simulink model "lab3_p9"  (R2020a)
settings: Solver=VariableStepAuto  StartTime=0.0  StopTime=mp.test_signal.duration  RelTol=1e-3
InitFcn:
  | sm_callback_init
StopFcn:
  | sm_callback_stop
values from neighbouring files (symbols this model uses):
  mp = sm_init_control_signals(mp)    [sm_callback_init.m]    (also in sm_callback_stop.m = sm_stop_verify(mp))
undefined symbols (not defined in the file or in its folder): magnitude
libraries: hdlsllib x9, simulink x3
settings Model: Creator=Owner  LastModifiedBy=Owner
settings DataIOCC: ReturnWorkspaceOutputs=off

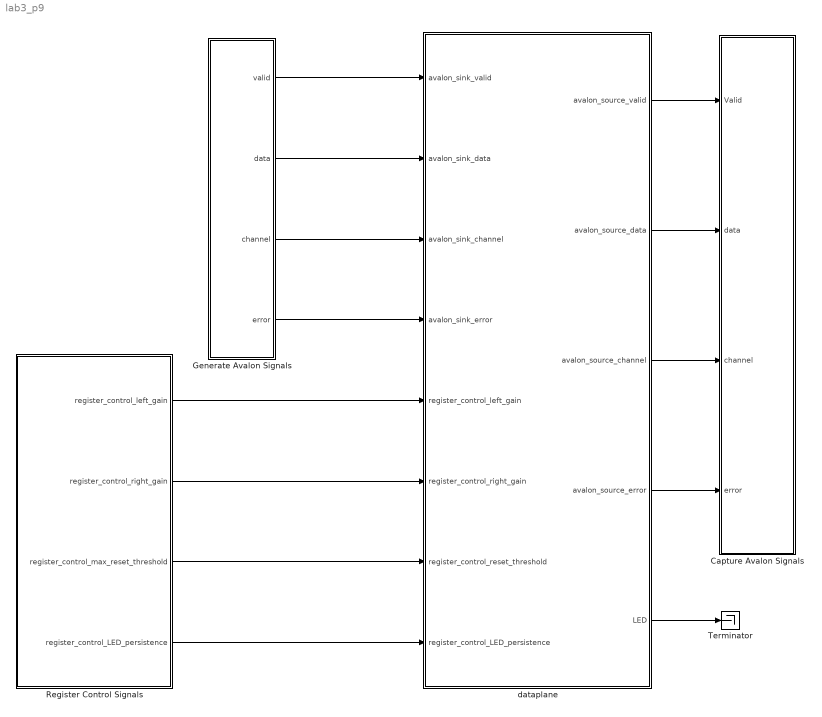
== system lab3_p9 ==
  Capture Avalon Signals : Subsystem
  Generate Avalon Signals : Subsystem
  Register Control Signals : Subsystem
  Terminator : Terminator
  dataplane : Subsystem
  wires:
  Generate Avalon Signals/1(valid) -> dataplane/1(avalon_sink_valid)
  Generate Avalon Signals/2(data) -> dataplane/2(avalon_sink_data)
  Generate Avalon Signals/3(channel) -> dataplane/3(avalon_sink_channel)
  Generate Avalon Signals/4(error) -> dataplane/4(avalon_sink_error)
  dataplane/1(avalon_source_valid) -> Capture Avalon Signals/1(Valid)
  dataplane/2(avalon_source_data) -> Capture Avalon Signals/2(data)
  dataplane/3(avalon_source_channel) -> Capture Avalon Signals/3(channel)
  dataplane/4(avalon_source_error) -> Capture Avalon Signals/4(error)
  Register Control Signals/2(register_control_right_gain) -> dataplane/6(register_control_right_gain)
  Register Control Signals/1(register_control_left_gain) -> dataplane/5(register_control_left_gain)
  Register Control Signals/3(register_control_max_reset_threshold) -> dataplane/7(register_control_reset_threshold)
  Register Control Signals/4(register_control_LED_persistence) -> dataplane/8(register_control_LED_persistence)
  dataplane/5(LED) -> Terminator/1

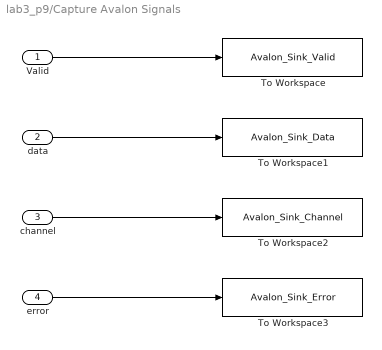
== system lab3_p9/Capture Avalon Signals ==
  Valid : Inport
  data : Inport  Port=2
  channel : Inport  Port=3
  error : Inport  Port=4
  To Workspace : ToWorkspace  VariableName=Avalon_Sink_Valid  SampleTime=-1
      settings: Save2DSignal=2-D array (concatenate along first dimension)
  To Workspace1 : ToWorkspace  VariableName=Avalon_Sink_Data  SampleTime=-1
      settings: Save2DSignal=2-D array (concatenate along first dimension)
  To Workspace2 : ToWorkspace  VariableName=Avalon_Sink_Channel  SampleTime=-1
      settings: Save2DSignal=2-D array (concatenate along first dimension)
  To Workspace3 : ToWorkspace  VariableName=Avalon_Sink_Error  SampleTime=-1
      settings: Save2DSignal=2-D array (concatenate along first dimension)
  wires:
  Valid/1 -> To Workspace/1
  data/1 -> To Workspace1/1
  channel/1 -> To Workspace2/1
  error/1 -> To Workspace3/1

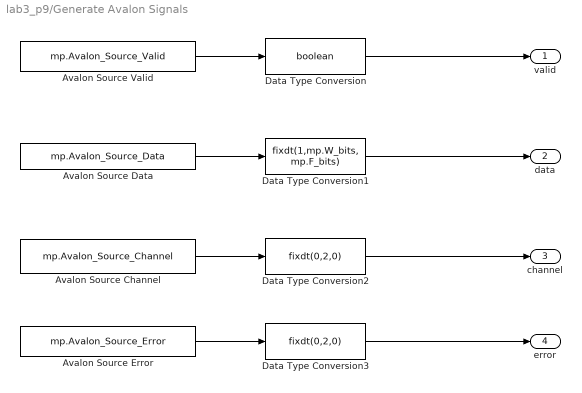
== system lab3_p9/Generate Avalon Signals ==
  Avalon Source Channel : FromWorkspace  VariableName=mp.Avalon_Source_Channel  OutDataTypeStr=double  SampleTime=mp.Ts_system
  Avalon Source Data : FromWorkspace  VariableName=mp.Avalon_Source_Data  OutDataTypeStr=double  SampleTime=mp.Ts_system
  Avalon Source Error : FromWorkspace  VariableName=mp.Avalon_Source_Error  OutDataTypeStr=double  SampleTime=mp.Ts_system
  Avalon Source Valid : FromWorkspace  VariableName=mp.Avalon_Source_Valid  OutDataTypeStr=double  SampleTime=mp.Ts_system
  Data Type Conversion : DataTypeConversion  OutDataTypeStr=boolean  RndMeth=Nearest
  Data Type Conversion1 : DataTypeConversion  OutDataTypeStr=fixdt(1,mp.W_bits, mp.F_bits)  RndMeth=Nearest
  Data Type Conversion2 : DataTypeConversion  OutDataTypeStr=fixdt(0,2,0)  RndMeth=Nearest
  Data Type Conversion3 : DataTypeConversion  OutDataTypeStr=fixdt(0,2,0)  RndMeth=Nearest
  valid : Outport
  data : Outport  Port=2
  channel : Outport  Port=3
  error : Outport  Port=4
  wires:
  Data Type Conversion/1 -> valid/1
  Avalon Source Valid/1 -> Data Type Conversion/1
  Avalon Source Data/1 -> Data Type Conversion1/1
  Data Type Conversion1/1 -> data/1
  Data Type Conversion2/1 -> channel/1
  Avalon Source Channel/1 -> Data Type Conversion2/1
  Data Type Conversion3/1 -> error/1
  Avalon Source Error/1 -> Data Type Conversion3/1

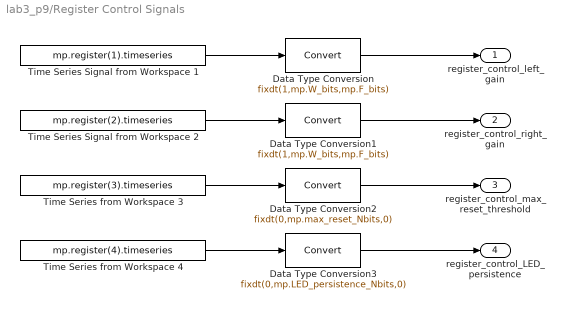
== system lab3_p9/Register Control Signals ==
  Data Type Conversion : DataTypeConversion  OutDataTypeStr=fixdt(1,mp.W_bits,mp.F_bits)
  Data Type Conversion1 : DataTypeConversion  OutDataTypeStr=fixdt(1,mp.W_bits,mp.F_bits)
  Data Type Conversion2 : DataTypeConversion  OutDataTypeStr=fixdt(0,mp.max_reset_Nbits,0)
  Data Type Conversion3 : DataTypeConversion  OutDataTypeStr=fixdt(0,mp.LED_persistence_Nbits,0)
  Time Series Signal from Workspace 1 : FromWorkspace  VariableName=mp.register(1).timeseries  OutDataTypeStr=double  SampleTime=mp.Ts_system
  Time Series Signal from Workspace 2 : FromWorkspace  VariableName=mp.register(2).timeseries  OutDataTypeStr=double  SampleTime=mp.Ts_system
  Time Series from Workspace 3 : FromWorkspace  VariableName=mp.register(3).timeseries  OutDataTypeStr=double  SampleTime=mp.Ts_system
  Time Series from Workspace 4 : FromWorkspace  VariableName=mp.register(4).timeseries  OutDataTypeStr=double  SampleTime=mp.Ts_system
  register_control_left_gain : Outport
  register_control_right_gain : Outport  Port=2
  register_control_max_reset_threshold : Outport  Port=3
  register_control_LED_persistence : Outport  Port=4
  wires:
  Time Series Signal from Workspace 1/1 -> Data Type Conversion/1
  Data Type Conversion/1 -> register_control_left_gain/1
  Time Series Signal from Workspace 2/1 -> Data Type Conversion1/1
  Data Type Conversion1/1 -> register_control_right_gain/1
  Data Type Conversion2/1 -> register_control_max_reset_threshold/1
  Data Type Conversion3/1 -> register_control_LED_persistence/1
  Time Series from Workspace 4/1 -> Data Type Conversion3/1
  Time Series from Workspace 3/1 -> Data Type Conversion2/1

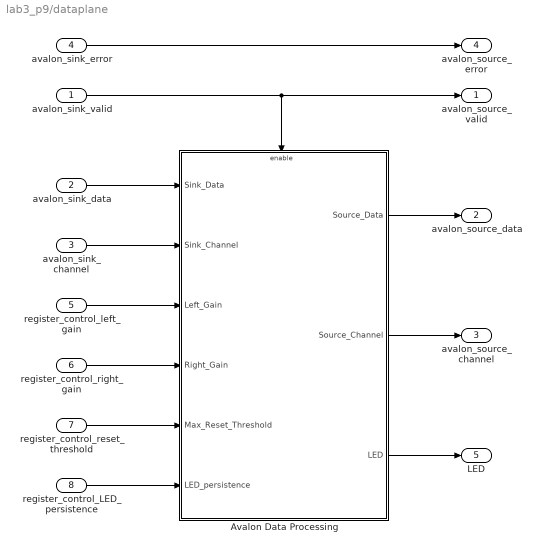
== system lab3_p9/dataplane ==
  avalon_sink_valid : Inport
  avalon_sink_data : Inport  Port=2
  avalon_sink_channel : Inport  Port=3
  avalon_sink_error : Inport  Port=4
  register_control_left_gain : Inport  Port=5
  register_control_right_gain : Inport  Port=6
  register_control_reset_threshold : Inport  Port=7
  register_control_LED_persistence : Inport  Port=8
  Avalon Data Processing : Subsystem  TreatAsAtomicUnit=on
  avalon_source_valid : Outport  VectorParamsAs1DForOutWhenUnconnected=off
  avalon_source_data : Outport  Port=2  VectorParamsAs1DForOutWhenUnconnected=off
  avalon_source_channel : Outport  Port=3  VectorParamsAs1DForOutWhenUnconnected=off
  avalon_source_error : Outport  Port=4  VectorParamsAs1DForOutWhenUnconnected=off
  LED : Outport  Port=5  VectorParamsAs1DForOutWhenUnconnected=off
  wires:
  avalon_sink_error/1 -> avalon_source_error/1
  avalon_sink_valid/1 -> avalon_source_valid/1, Avalon Data Processing/Enable
  Avalon Data Processing/1(Source_Data) -> avalon_source_data/1
  Avalon Data Processing/2(Source_Channel) -> avalon_source_channel/1
  avalon_sink_data/1 -> Avalon Data Processing/1(Sink_Data)
  avalon_sink_channel/1 -> Avalon Data Processing/2(Sink_Channel)
  register_control_right_gain/1 -> Avalon Data Processing/4(Right_Gain)
  register_control_left_gain/1 -> Avalon Data Processing/3(Left_Gain)
  register_control_reset_threshold/1 -> Avalon Data Processing/5(Max_Reset_Threshold)
  register_control_LED_persistence/1 -> Avalon Data Processing/6(LED_persistence)
  Avalon Data Processing/3(LED) -> LED/1

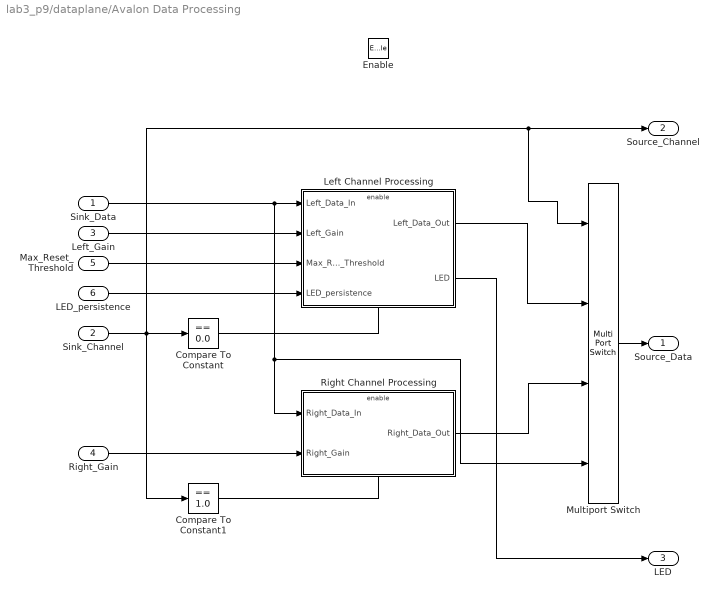
== system lab3_p9/dataplane/Avalon Data Processing ==
  Sink_Data : Inport
  Sink_Channel : Inport  Port=2
  Left_Gain : Inport  Port=3
  Right_Gain : Inport  Port=4
  Max_Reset_Threshold : Inport  Port=5
  LED_persistence : Inport  Port=6
  Enable : EnablePort
  Compare To Constant : simulink/Logic and Bit Operations/Compare To Constant  relop===  const=0.0  OutDataTypeStr=boolean
  Compare To Constant1 : simulink/Logic and Bit Operations/Compare To Constant  relop===  const=1.0  OutDataTypeStr=boolean
  Left Channel Processing : Subsystem  TreatAsAtomicUnit=on
  Multiport Switch : MultiPortSwitch  DataPortOrder=Zero-based contiguous  zeroidx=on
  Right Channel Processing : Subsystem  TreatAsAtomicUnit=on
  Source_Data : Outport
  Source_Channel : Outport  Port=2
  LED : Outport  Port=3
  wires:
  Sink_Data/1 -> Multiport Switch/4, Right Channel Processing/1(Right_Data_In), Left Channel Processing/1(Left_Data_In)
  Sink_Channel/1 -> Compare To Constant1/1, Multiport Switch/1, Source_Channel/1, Compare To Constant/1
  Left_Gain/1 -> Left Channel Processing/2(Left_Gain)
  Right_Gain/1 -> Right Channel Processing/2(Right_Gain)
  Compare To Constant1/1 -> Right Channel Processing/Enable
  Compare To Constant/1 -> Left Channel Processing/Enable
  Multiport Switch/1 -> Source_Data/1
  Left Channel Processing/1(Left_Data_Out) -> Multiport Switch/2
  Right Channel Processing/1(Right_Data_Out) -> Multiport Switch/3
  Left Channel Processing/2(LED) -> LED/1
  LED_persistence/1 -> Left Channel Processing/4(LED_persistence)
  Max_Reset_Threshold/1 -> Left Channel Processing/3(Max_Reset_Threshold)

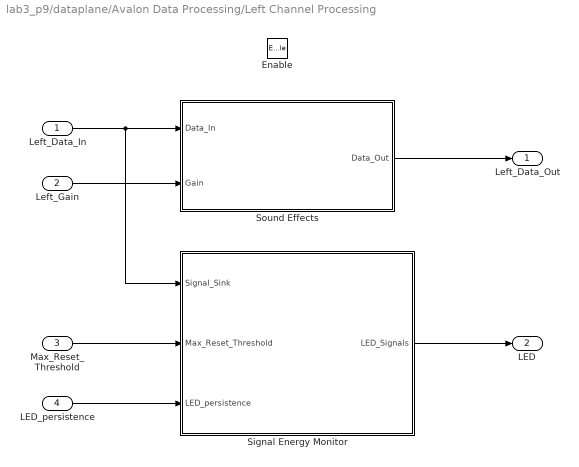
== system lab3_p9/dataplane/Avalon Data Processing/Left Channel Processing ==
  Left_Data_In : Inport
  Left_Gain : Inport  Port=2
  Max_Reset_Threshold : Inport  Port=3
  LED_persistence : Inport  Port=4
  Enable : EnablePort
  Signal Energy Monitor : Subsystem
  Sound Effects : Subsystem
  Left_Data_Out : Outport  InitialOutput=0  VectorParamsAs1DForOutWhenUnconnected=off
  LED : Outport  Port=2  InitialOutput=0  VectorParamsAs1DForOutWhenUnconnected=off
  wires:
  Sound Effects/1(Data_Out) -> Left_Data_Out/1
  Left_Gain/1 -> Sound Effects/2(Gain)
  Signal Energy Monitor/1(LED_Signals) -> LED/1
  LED_persistence/1 -> Signal Energy Monitor/3(LED_persistence)
  Left_Data_In/1 -> Signal Energy Monitor/1(Signal_Sink), Sound Effects/1(Data_In)
  Max_Reset_Threshold/1 -> Signal Energy Monitor/2(Max_Reset_Threshold)

== system lab3_p9/dataplane/Avalon Data Processing/Right Channel Processing ==
  Right_Data_In : Inport
  Right_Gain : Inport  Port=2
  Enable : EnablePort
  Sound Effects : Subsystem
  Right_Data_Out : Outport  InitialOutput=0  VectorParamsAs1DForOutWhenUnconnected=off
  wires:
  Right_Data_In/1 -> Sound Effects/1(Data_In)
  Right_Gain/1 -> Sound Effects/2(Gain)
  Sound Effects/1(Data_Out) -> Right_Data_Out/1

== system lab3_p9/dataplane/Avalon Data Processing/Left Channel Processing/Signal Energy Monitor ==
  Signal_Sink : Inport
  Max_Reset_Threshold : Inport  Port=2
  LED_persistence : Inport  Port=3
  LED_Driver : Subsystem
  Normalize Signal : Subsystem
  LED_Signals : Outport  VectorParamsAs1DForOutWhenUnconnected=off
  wires:
  Signal_Sink/1 -> Normalize Signal/1(Signal_Sink)
  Max_Reset_Threshold/1 -> Normalize Signal/2(Max_Reset_Threshold)
  Normalize Signal/1(Normalized_Signal_Energy) -> LED_Driver/1(Normalized_Signal)
  LED_Driver/1(LED_Signals) -> LED_Signals/1
  LED_persistence/1 -> LED_Driver/2(LED_persistence)

== system lab3_p9/dataplane/Avalon Data Processing/Left Channel Processing/Sound Effects ==
  Data_In : Inport
  Gain : Inport  Port=2
  Data Type Conversion : DataTypeConversion  OutDataTypeStr=fixdt(1,mp.W_bits,mp.F_bits)  RndMeth=Nearest
  Product : Product
  Data_Out : Outport
  wires:
  Product/1 -> Data Type Conversion/1
  Gain/1 -> Product/2
  Data_In/1 -> Product/1
  Data Type Conversion/1 -> Data_Out/1

== system lab3_p9/dataplane/Avalon Data Processing/Right Channel Processing/Sound Effects ==
  Data_In : Inport
  Gain : Inport  Port=2
  Data Type Conversion : DataTypeConversion  OutDataTypeStr=fixdt(1,mp.W_bits,mp.F_bits)  RndMeth=Nearest
  Product : Product
  Data_Out : Outport
  wires:
  Product/1 -> Data Type Conversion/1
  Gain/1 -> Product/2
  Data_In/1 -> Product/1
  Data Type Conversion/1 -> Data_Out/1

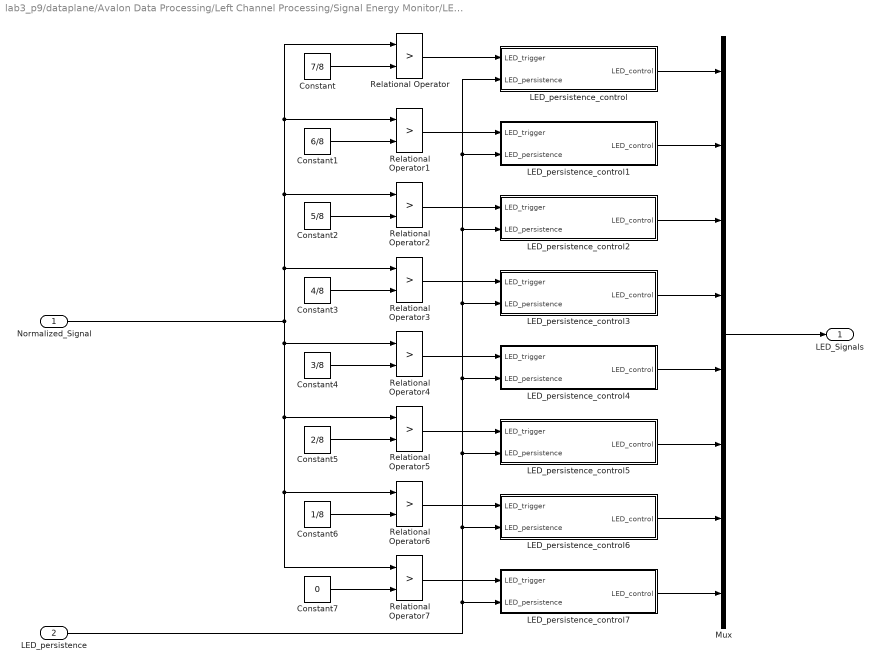
== system lab3_p9/dataplane/Avalon Data Processing/Left Channel Processing/Signal Energy Monitor/LED_Driver ==
  Normalized_Signal : Inport
  LED_persistence : Inport  Port=2
  Constant : Constant  Value=7/8  OutDataTypeStr=fixdt(1,mp.W_bits,mp.F_bits)  SampleTime=mp.Ts_system
  Constant1 : Constant  Value=6/8  OutDataTypeStr=fixdt(1,mp.W_bits,mp.F_bits)  SampleTime=mp.Ts_system
  Constant2 : Constant  Value=5/8  OutDataTypeStr=fixdt(1,mp.W_bits,mp.F_bits)  SampleTime=mp.Ts_system
  Constant3 : Constant  Value=4/8  OutDataTypeStr=fixdt(1,mp.W_bits,mp.F_bits)  SampleTime=mp.Ts_system
  Constant4 : Constant  Value=3/8  OutDataTypeStr=fixdt(1,mp.W_bits,mp.F_bits)  SampleTime=mp.Ts_system
  Constant5 : Constant  Value=2/8  OutDataTypeStr=fixdt(1,mp.W_bits,mp.F_bits)  SampleTime=mp.Ts_system
  Constant6 : Constant  Value=1/8  OutDataTypeStr=fixdt(1,mp.W_bits,mp.F_bits)  SampleTime=mp.Ts_system
  Constant7 : Constant  Value=0  OutDataTypeStr=fixdt(1,mp.W_bits,mp.F_bits)  SampleTime=mp.Ts_system
  LED_persistence_control : Subsystem
  LED_persistence_control1 : Subsystem
  LED_persistence_control2 : Subsystem
  LED_persistence_control3 : Subsystem
  LED_persistence_control4 : Subsystem
  LED_persistence_control5 : Subsystem
  LED_persistence_control6 : Subsystem
  LED_persistence_control7 : Subsystem
  Mux : Mux  Inputs=8
  Relational Operator{,1..7} (8 alike) : RelationalOperator  Operator=>  OutDataTypeStr=boolean  RndMeth=Nearest
  LED_Signals : Outport
  wires:
  Constant/1 -> Relational Operator/2
  Normalized_Signal/1 -> Relational Operator4/1, Relational Operator5/1, Relational Operator7/1, Relational Operator6/1, Relational Operator/1, Relational Operator1/1, Relational Operator2/1, Relational Operator3/1
  Constant1/1 -> Relational Operator1/2
  Constant2/1 -> Relational Operator2/2
  Constant3/1 -> Relational Operator3/2
  Constant4/1 -> Relational Operator4/2
  Constant5/1 -> Relational Operator5/2
  Constant6/1 -> Relational Operator6/2
  Constant7/1 -> Relational Operator7/2
  Mux/1 -> LED_Signals/1
  Relational Operator/1 -> LED_persistence_control/1(LED_trigger)
  LED_persistence_control/1(LED_control) -> Mux/1
  Relational Operator1/1 -> LED_persistence_control1/1(LED_trigger)
  Relational Operator2/1 -> LED_persistence_control2/1(LED_trigger)
  Relational Operator3/1 -> LED_persistence_control3/1(LED_trigger)
  Relational Operator4/1 -> LED_persistence_control4/1(LED_trigger)
  Relational Operator5/1 -> LED_persistence_control5/1(LED_trigger)
  LED_persistence/1 -> LED_persistence_control7/2(LED_persistence), LED_persistence_control6/2(LED_persistence), LED_persistence_control5/2(LED_persistence), LED_persistence_control4/2(LED_persistence), LED_persistence_control3/2(LED_persistence), LED_persistence_control2/2(LED_persistence), LED_persistence_control1/2(LED_persistence), LED_persistence_control/2(LED_persistence)
  Relational Operator6/1 -> LED_persistence_control6/1(LED_trigger)
  Relational Operator7/1 -> LED_persistence_control7/1(LED_trigger)
  LED_persistence_control7/1(LED_control) -> Mux/8
  LED_persistence_control6/1(LED_control) -> Mux/7
  LED_persistence_control5/1(LED_control) -> Mux/6
  LED_persistence_control4/1(LED_control) -> Mux/5
  LED_persistence_control3/1(LED_control) -> Mux/4
  LED_persistence_control2/1(LED_control) -> Mux/3
  LED_persistence_control1/1(LED_control) -> Mux/2

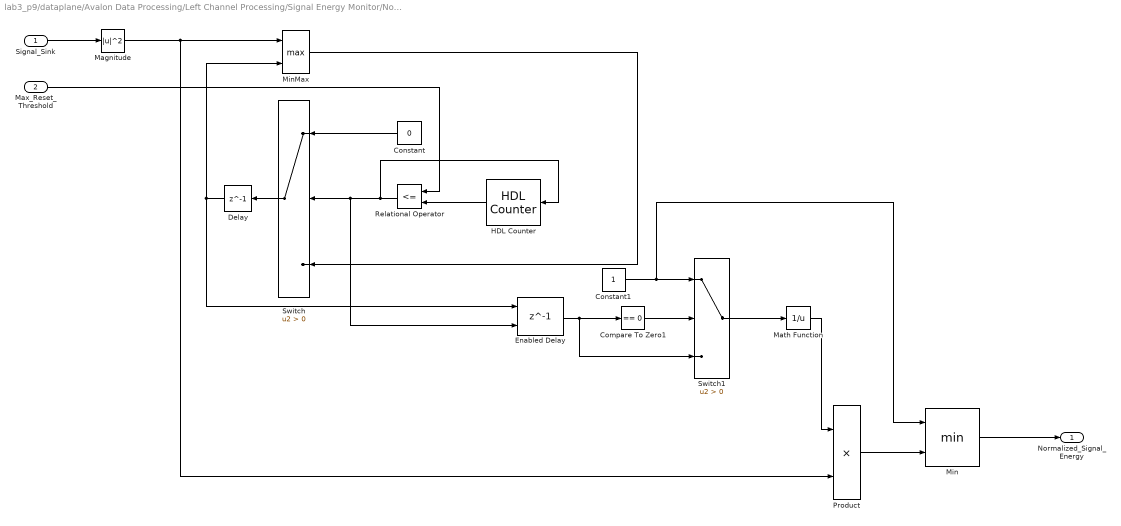
== system lab3_p9/dataplane/Avalon Data Processing/Left Channel Processing/Signal Energy Monitor/Normalize Signal ==
  Signal_Sink : Inport
  Max_Reset_Threshold : Inport  Port=2
  Compare To Zero1 : simulink/Logic and Bit Operations/Compare To Zero  relop===  OutDataTypeStr=boolean
  Constant : Constant  Value=0  OutDataTypeStr=fixdt(1,mp.W_bits,mp.F_bits)  SampleTime=mp.Ts_system
  Constant1 : Constant  OutDataTypeStr=fixdt(1,mp.W_bits,mp.F_bits)  SampleTime=mp.Ts_system
  Delay : Delay  DelayLength=1
  Enabled Delay : Delay  DelayLength=1  ShowEnablePort=on
      settings: InputPortMap=u0,e6
  HDL Counter : hdlsllib/Sources/HDL Counter  CountType=Free running  CountInit=0  CountStep=1  CountMax=25  CountFromType=Initial value  CountFrom=0  CountResetPort=on  CountLoadPort=off  CountEnbPort=off  CountDirPort=off  CountDataType=Unsigned  CountWordLen=mp.max_reset_Nbits  CountFracLen=0  CountSampTime=1
  Magnitude : Math  Operator=magnitude^2  SignedPower=on  RndMeth=Zero  SaturateOnIntegerOverflow=on
  Math Function : Math  Operator=reciprocal  OutDataTypeStr=fixdt(1,32,24)  SaturateOnIntegerOverflow=on
  Min : MinMax  Inputs=2  OutDataTypeStr=fixdt(1,mp.W_bits,mp.F_bits)
  MinMax : MinMax  Function=max  Inputs=2
  Product : Product  OutDataTypeStr=fixdt(1,mp.W_bits,mp.F_bits)
  Relational Operator : RelationalOperator  Operator=<=  OutDataTypeStr=boolean  RndMeth=Nearest
  Switch : Switch  Criteria=u2 > Threshold
  Switch1 : Switch  Criteria=u2 > Threshold
  Normalized_Signal_Energy : Outport
  wires:
  Delay/1 -> Enabled Delay/1, MinMax/2
  Enabled Delay/1 -> Switch1/3, Compare To Zero1/1
  Min/1 -> Normalized_Signal_Energy/1
  Math Function/1 -> Product/1
  Relational Operator/1 -> HDL Counter/1, Enabled Delay/2, Switch/2
  Constant/1 -> Switch/1
  MinMax/1 -> Switch/3
  Constant1/1 -> Min/1, Switch1/1
  Compare To Zero1/1 -> Switch1/2
  Magnitude/1 -> Product/2, MinMax/1
  Switch/1 -> Delay/1
  Signal_Sink/1 -> Magnitude/1
  Switch1/1 -> Math Function/1
  Product/1 -> Min/2
  HDL Counter/1 -> Relational Operator/2
  Max_Reset_Threshold/1 -> Relational Operator/1

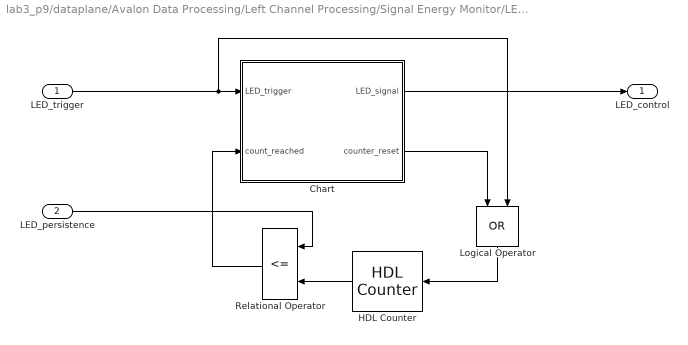
== system lab3_p9/dataplane/Avalon Data Processing/Left Channel Processing/Signal Energy Monitor/LED_Driver/LED_persistence_control ==
  LED_trigger : Inport
  LED_persistence : Inport  Port=2
  Chart : Stateflow chart  TreatAsAtomicUnit=on
  HDL Counter : hdlsllib/Sources/HDL Counter  CountType=Free running  CountInit=0  CountStep=1  CountMax=25  CountFromType=Initial value  CountFrom=0  CountResetPort=on  CountLoadPort=off  CountEnbPort=off  CountDirPort=off  CountDataType=Unsigned  CountWordLen=mp.LED_persistence_Nbits  CountFracLen=0  CountSampTime=1
  Logical Operator : Logic  Operator=OR  AllPortsSameDT=off  OutDataTypeStr=boolean
  Relational Operator : RelationalOperator  Operator=<=  OutDataTypeStr=boolean  RndMeth=Nearest
  LED_control : Outport
  wires:
  LED_trigger/1 -> Logical Operator/2, Chart/1(LED_trigger)
  Logical Operator/1 -> HDL Counter/1
  Chart/2(counter_reset) -> Logical Operator/1
  LED_persistence/1 -> Relational Operator/1
  HDL Counter/1 -> Relational Operator/2
  Relational Operator/1 -> Chart/2(count_reached)
  Chart/1(LED_signal) -> LED_control/1

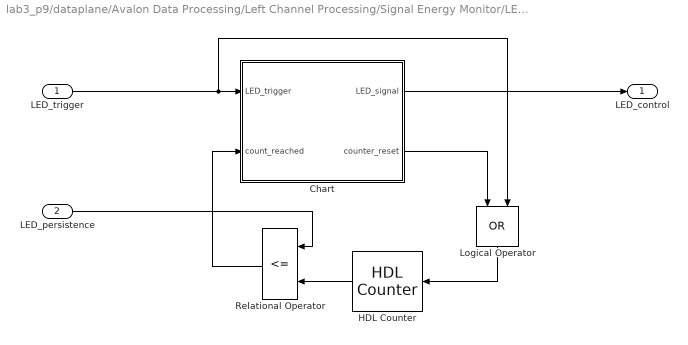
== system lab3_p9/dataplane/Avalon Data Processing/Left Channel Processing/Signal Energy Monitor/LED_Driver/LED_persistence_control1 ==
  LED_trigger : Inport
  LED_persistence : Inport  Port=2
  Chart : Stateflow chart  TreatAsAtomicUnit=on
  HDL Counter : hdlsllib/Sources/HDL Counter  CountType=Free running  CountInit=0  CountStep=1  CountMax=25  CountFromType=Initial value  CountFrom=0  CountResetPort=on  CountLoadPort=off  CountEnbPort=off  CountDirPort=off  CountDataType=Unsigned  CountWordLen=mp.LED_persistence_Nbits  CountFracLen=0  CountSampTime=1
  Logical Operator : Logic  Operator=OR  AllPortsSameDT=off  OutDataTypeStr=boolean
  Relational Operator : RelationalOperator  Operator=<=  OutDataTypeStr=boolean  RndMeth=Nearest
  LED_control : Outport
  wires:
  LED_trigger/1 -> Logical Operator/2, Chart/1(LED_trigger)
  Logical Operator/1 -> HDL Counter/1
  Chart/2(counter_reset) -> Logical Operator/1
  LED_persistence/1 -> Relational Operator/1
  HDL Counter/1 -> Relational Operator/2
  Relational Operator/1 -> Chart/2(count_reached)
  Chart/1(LED_signal) -> LED_control/1

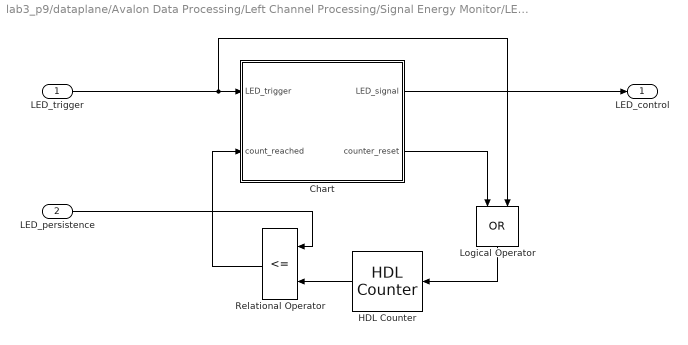
== system lab3_p9/dataplane/Avalon Data Processing/Left Channel Processing/Signal Energy Monitor/LED_Driver/LED_persistence_control2 ==
  LED_trigger : Inport
  LED_persistence : Inport  Port=2
  Chart : Stateflow chart  TreatAsAtomicUnit=on
  HDL Counter : hdlsllib/Sources/HDL Counter  CountType=Free running  CountInit=0  CountStep=1  CountMax=25  CountFromType=Initial value  CountFrom=0  CountResetPort=on  CountLoadPort=off  CountEnbPort=off  CountDirPort=off  CountDataType=Unsigned  CountWordLen=mp.LED_persistence_Nbits  CountFracLen=0  CountSampTime=1
  Logical Operator : Logic  Operator=OR  AllPortsSameDT=off  OutDataTypeStr=boolean
  Relational Operator : RelationalOperator  Operator=<=  OutDataTypeStr=boolean  RndMeth=Nearest
  LED_control : Outport
  wires:
  LED_trigger/1 -> Logical Operator/2, Chart/1(LED_trigger)
  Logical Operator/1 -> HDL Counter/1
  Chart/2(counter_reset) -> Logical Operator/1
  LED_persistence/1 -> Relational Operator/1
  HDL Counter/1 -> Relational Operator/2
  Relational Operator/1 -> Chart/2(count_reached)
  Chart/1(LED_signal) -> LED_control/1

== system lab3_p9/dataplane/Avalon Data Processing/Left Channel Processing/Signal Energy Monitor/LED_Driver/LED_persistence_control3 ==
  LED_trigger : Inport
  LED_persistence : Inport  Port=2
  Chart : Stateflow chart  TreatAsAtomicUnit=on
  HDL Counter : hdlsllib/Sources/HDL Counter  CountType=Free running  CountInit=0  CountStep=1  CountMax=25  CountFromType=Initial value  CountFrom=0  CountResetPort=on  CountLoadPort=off  CountEnbPort=off  CountDirPort=off  CountDataType=Unsigned  CountWordLen=mp.LED_persistence_Nbits  CountFracLen=0  CountSampTime=1
  Logical Operator : Logic  Operator=OR  AllPortsSameDT=off  OutDataTypeStr=boolean
  Relational Operator : RelationalOperator  Operator=<=  OutDataTypeStr=boolean  RndMeth=Nearest
  LED_control : Outport
  wires:
  LED_trigger/1 -> Logical Operator/2, Chart/1(LED_trigger)
  Logical Operator/1 -> HDL Counter/1
  Chart/2(counter_reset) -> Logical Operator/1
  LED_persistence/1 -> Relational Operator/1
  HDL Counter/1 -> Relational Operator/2
  Relational Operator/1 -> Chart/2(count_reached)
  Chart/1(LED_signal) -> LED_control/1

== system lab3_p9/dataplane/Avalon Data Processing/Left Channel Processing/Signal Energy Monitor/LED_Driver/LED_persistence_control4 ==
  LED_trigger : Inport
  LED_persistence : Inport  Port=2
  Chart : Stateflow chart  TreatAsAtomicUnit=on
  HDL Counter : hdlsllib/Sources/HDL Counter  CountType=Free running  CountInit=0  CountStep=1  CountMax=25  CountFromType=Initial value  CountFrom=0  CountResetPort=on  CountLoadPort=off  CountEnbPort=off  CountDirPort=off  CountDataType=Unsigned  CountWordLen=mp.LED_persistence_Nbits  CountFracLen=0  CountSampTime=1
  Logical Operator : Logic  Operator=OR  AllPortsSameDT=off  OutDataTypeStr=boolean
  Relational Operator : RelationalOperator  Operator=<=  OutDataTypeStr=boolean  RndMeth=Nearest
  LED_control : Outport
  wires:
  LED_trigger/1 -> Logical Operator/2, Chart/1(LED_trigger)
  Logical Operator/1 -> HDL Counter/1
  Chart/2(counter_reset) -> Logical Operator/1
  LED_persistence/1 -> Relational Operator/1
  HDL Counter/1 -> Relational Operator/2
  Relational Operator/1 -> Chart/2(count_reached)
  Chart/1(LED_signal) -> LED_control/1

== system lab3_p9/dataplane/Avalon Data Processing/Left Channel Processing/Signal Energy Monitor/LED_Driver/LED_persistence_control5 ==
  LED_trigger : Inport
  LED_persistence : Inport  Port=2
  Chart : Stateflow chart  TreatAsAtomicUnit=on
  HDL Counter : hdlsllib/Sources/HDL Counter  CountType=Free running  CountInit=0  CountStep=1  CountMax=25  CountFromType=Initial value  CountFrom=0  CountResetPort=on  CountLoadPort=off  CountEnbPort=off  CountDirPort=off  CountDataType=Unsigned  CountWordLen=mp.LED_persistence_Nbits  CountFracLen=0  CountSampTime=1
  Logical Operator : Logic  Operator=OR  AllPortsSameDT=off  OutDataTypeStr=boolean
  Relational Operator : RelationalOperator  Operator=<=  OutDataTypeStr=boolean  RndMeth=Nearest
  LED_control : Outport
  wires:
  LED_trigger/1 -> Logical Operator/2, Chart/1(LED_trigger)
  Logical Operator/1 -> HDL Counter/1
  Chart/2(counter_reset) -> Logical Operator/1
  LED_persistence/1 -> Relational Operator/1
  HDL Counter/1 -> Relational Operator/2
  Relational Operator/1 -> Chart/2(count_reached)
  Chart/1(LED_signal) -> LED_control/1

== system lab3_p9/dataplane/Avalon Data Processing/Left Channel Processing/Signal Energy Monitor/LED_Driver/LED_persistence_control6 ==
  LED_trigger : Inport
  LED_persistence : Inport  Port=2
  Chart : Stateflow chart  TreatAsAtomicUnit=on
  HDL Counter : hdlsllib/Sources/HDL Counter  CountType=Free running  CountInit=0  CountStep=1  CountMax=25  CountFromType=Initial value  CountFrom=0  CountResetPort=on  CountLoadPort=off  CountEnbPort=off  CountDirPort=off  CountDataType=Unsigned  CountWordLen=mp.LED_persistence_Nbits  CountFracLen=0  CountSampTime=1
  Logical Operator : Logic  Operator=OR  AllPortsSameDT=off  OutDataTypeStr=boolean
  Relational Operator : RelationalOperator  Operator=<=  OutDataTypeStr=boolean  RndMeth=Nearest
  LED_control : Outport
  wires:
  LED_trigger/1 -> Logical Operator/2, Chart/1(LED_trigger)
  Logical Operator/1 -> HDL Counter/1
  Chart/2(counter_reset) -> Logical Operator/1
  LED_persistence/1 -> Relational Operator/1
  HDL Counter/1 -> Relational Operator/2
  Relational Operator/1 -> Chart/2(count_reached)
  Chart/1(LED_signal) -> LED_control/1

== system lab3_p9/dataplane/Avalon Data Processing/Left Channel Processing/Signal Energy Monitor/LED_Driver/LED_persistence_control7 ==
  LED_trigger : Inport
  LED_persistence : Inport  Port=2
  Chart : Stateflow chart  TreatAsAtomicUnit=on
  HDL Counter : hdlsllib/Sources/HDL Counter  CountType=Free running  CountInit=0  CountStep=1  CountMax=25  CountFromType=Initial value  CountFrom=0  CountResetPort=on  CountLoadPort=off  CountEnbPort=off  CountDirPort=off  CountDataType=Unsigned  CountWordLen=mp.LED_persistence_Nbits  CountFracLen=0  CountSampTime=1
  Logical Operator : Logic  Operator=OR  AllPortsSameDT=off  OutDataTypeStr=boolean
  Relational Operator : RelationalOperator  Operator=<=  OutDataTypeStr=boolean  RndMeth=Nearest
  LED_control : Outport
  wires:
  LED_trigger/1 -> Logical Operator/2, Chart/1(LED_trigger)
  Logical Operator/1 -> HDL Counter/1
  Chart/2(counter_reset) -> Logical Operator/1
  LED_persistence/1 -> Relational Operator/1
  HDL Counter/1 -> Relational Operator/2
  Relational Operator/1 -> Chart/2(count_reached)
  Chart/1(LED_signal) -> LED_control/1

== stateflow chart lab3_p9/dataplane/Avalon Data Processing/Left Channel Processing/Signal Energy Monitor/LED_Driver/LED_persistence_control1/Chart ==
  state LED_off
    entry: LED_signal=false;
    entry: counter_reset=true;
  state LED_on
    entry: LED_signal=true;
    entry: counter_reset=false;
  (default) -> LED_off
  LED_off -> LED_on : [LED_trigger==1]
  LED_on -> LED_off : [count_reached==1]
  data: LED_trigger input; count_reached input; LED_signal output; counter_reset output

== stateflow chart lab3_p9/dataplane/Avalon Data Processing/Left Channel Processing/Signal Energy Monitor/LED_Driver/LED_persistence_control2/Chart ==
  state LED_off
    entry: LED_signal=false;
    entry: counter_reset=true;
  state LED_on
    entry: LED_signal=true;
    entry: counter_reset=false;
  (default) -> LED_off
  LED_off -> LED_on : [LED_trigger==1]
  LED_on -> LED_off : [count_reached==1]
  data: LED_trigger input; count_reached input; LED_signal output; counter_reset output

== stateflow chart lab3_p9/dataplane/Avalon Data Processing/Left Channel Processing/Signal Energy Monitor/LED_Driver/LED_persistence_control/Chart ==
  state LED_off
    entry: LED_signal=false;
    entry: counter_reset=true;
  state LED_on
    entry: LED_signal=true;
    entry: counter_reset=false;
  (default) -> LED_off
  LED_off -> LED_on : [LED_trigger==1]
  LED_on -> LED_off : [count_reached==1]
  data: LED_trigger input; count_reached input; LED_signal output; counter_reset output

== stateflow chart lab3_p9/dataplane/Avalon Data Processing/Left Channel Processing/Signal Energy Monitor/LED_Driver/LED_persistence_control3/Chart ==
  state LED_off
    entry: LED_signal=false;
    entry: counter_reset=true;
  state LED_on
    entry: LED_signal=true;
    entry: counter_reset=false;
  (default) -> LED_off
  LED_off -> LED_on : [LED_trigger==1]
  LED_on -> LED_off : [count_reached==1]
  data: LED_trigger input; count_reached input; LED_signal output; counter_reset output

== stateflow chart lab3_p9/dataplane/Avalon Data Processing/Left Channel Processing/Signal Energy Monitor/LED_Driver/LED_persistence_control4/Chart ==
  state LED_off
    entry: LED_signal=false;
    entry: counter_reset=true;
  state LED_on
    entry: LED_signal=true;
    entry: counter_reset=false;
  (default) -> LED_off
  LED_off -> LED_on : [LED_trigger==1]
  LED_on -> LED_off : [count_reached==1]
  data: LED_trigger input; count_reached input; LED_signal output; counter_reset output

== stateflow chart lab3_p9/dataplane/Avalon Data Processing/Left Channel Processing/Signal Energy Monitor/LED_Driver/LED_persistence_control5/Chart ==
  state LED_off
    entry: LED_signal=false;
    entry: counter_reset=true;
  state LED_on
    entry: LED_signal=true;
    entry: counter_reset=false;
  (default) -> LED_off
  LED_off -> LED_on : [LED_trigger==1]
  LED_on -> LED_off : [count_reached==1]
  data: LED_trigger input; count_reached input; LED_signal output; counter_reset output

== stateflow chart lab3_p9/dataplane/Avalon Data Processing/Left Channel Processing/Signal Energy Monitor/LED_Driver/LED_persistence_control6/Chart ==
  state LED_off
    entry: LED_signal=false;
    entry: counter_reset=true;
  state LED_on
    entry: LED_signal=true;
    entry: counter_reset=false;
  (default) -> LED_off
  LED_off -> LED_on : [LED_trigger==1]
  LED_on -> LED_off : [count_reached==1]
  data: LED_trigger input; count_reached input; LED_signal output; counter_reset output

== stateflow chart lab3_p9/dataplane/Avalon Data Processing/Left Channel Processing/Signal Energy Monitor/LED_Driver/LED_persistence_control7/Chart ==
  state LED_off
    entry: LED_signal=false;
    entry: counter_reset=true;
  state LED_on
    entry: LED_signal=true;
    entry: counter_reset=false;
  (default) -> LED_off
  LED_off -> LED_on : [LED_trigger==1]
  LED_on -> LED_off : [count_reached==1]
  data: LED_trigger input; count_reached input; LED_signal output; counter_reset output
